simulink model "Mdl4ws_TS8"  (Simulink 5.0)
settings: Solver=ode45  SolverMode=SingleTasking  StartTime=0  StopTime=15  FixedStep=0.002  RelTol=1e-3  AbsTol=1e-6
libraries: Solver_SF x1
settings Model: LastModifiedBy=ywata  ExtModeTrigMode=oneshot  ExtModeArmWhenConnect=off  LimitDataPoints=off  SignalLoggingName=logsout  BlockReductionOpt=off  BooleanDataType=off  RTWTemplateMakefile=grt_vc.tmf  RTWOptions="-aEnforceIntegerDowncast=1 -aFoldNonRolledExpr=1 -aInlineInvariantSignals=0 -aInlineParameters=0 -aLocalBlockOutputs=1 -aRollThreshold=5 -aGenerateReport=0 -aGenCodeOnly=0 -aRTWVerbose=1 -aIncludeHyperlinkInReport=0 -aLaunchReport=0 -aForceParamTrailComments=0 -aGenerateComments=1 -aIgnoreCustomStorageClasses=1 -aIncHierarchyInIds=0 -aMaxRTWIdLen=31 -aShowEliminatedStatements=0 -aPrefixModelToSubsysFcnNames=1 -aIncDataTypeInIds=0 -aInsertBlockDesc=0 -aSimulinkBlockComments=1 -aInlinedPrmAccess=\"Literals\"  -aSuppressErrorStatus=0 -aModelReferenceCompliant=1 -aSupportNonInlinedSFcns=1 -aSupportContinuousTime=1 -aSupportComplex=1 -aSupportNonFinite=1 -aSupportAbsoluteTime=1 -aTargetPreCompLibLocation=\"\" -aTargetLibSuffix=\"\" -aTargetFcnLib=\"ansi_tfl_tmw.mat\" -aMultiInstanceERTCode=0 -aLogVarNameModifier=\"rt_\" -aIsPILTarget=0 -aCombineOutputUpdateFcns=0 -aGenerateASAP2=0 -aGenerateSampleERTMain=0 -aGenerateFullHeader=1 -aUtilityFuncGeneration=\"Auto\" -aIncludeFileDelimiter=\"Auto\" -aIncludeMdlTerminateFcn=1 -aPurelyIntegerCode=0 -aERTCustomFileBanners=0 -aRTWCAPIStates=0 -aRTWCAPIParams=0 -aRTWCAPISignals=0 -aMatFileLogging=1 -aGenFloatMathFcnCalls=\"ANSI_C\" -aExtModeMexFile=\"ext_comm\" -aExtModeTransport=0 -aExtModeStaticAllocSize=1000000 -aExtModeTesting=0 -aExtModeStaticAlloc=0 -aExtMode=0"

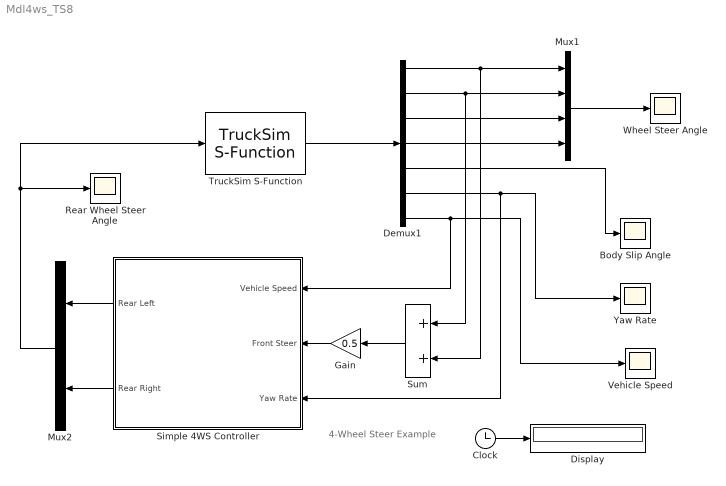
== system Mdl4ws_TS8 ==
  note: 4-Wheel Steer Example
  Body Slip Angle : Scope
      settings: TickLabels=on  YMin=-1  YMax=1.5  DataFormat=Array  Decimation=10
  Clock : Clock
      settings: Decimation=10
  Demux1 : Demux  Outputs=[1 1 1 1 1 1 1]
  Display : Display
      settings: Format=bank  Decimation=100
  Gain : Gain  Orientation=left  Gain=0.5  SaturateOnIntegerOverflow=on
  Mux1 : Mux
  Mux2 : Mux  Orientation=left  Inputs=2
  Rear Wheel Steer Angle : Scope
      settings: TickLabels=on  YMin=-2  YMax=2  DataFormat=Array  Decimation=10
  Simple 4WS Controller : Subsystem  Orientation=left  mask{m=7960, lf=3.102, lr=1.388, Cf=162521, Cr=139081}
      mask prompts: m "body mass (kg)"; lf "length f-G (m)"; lr "length r-G (m)"; Cf "conering power f  (N/rad)"; Cr "conering power r  (N/rad)"
  Sum : Sum  Orientation=left  SaturateOnIntegerOverflow=on  InputSameDT=on
  TruckSim S-Function : Solver_SF/TruckSim S-Function  Priority=1  AncestorBlock=Solver_SF/CarSim S-Function  VehicleCode=???
      settings: AttributesFormatString=Vehicle Code: %<VehicleCode>
  Vehicle Speed : Scope
      settings: TickLabels=on  TimeRange=12  YMin=99.5  YMax=100.5  DataFormat=Array  Decimation=10
  Wheel Steer Angle : Scope
      settings: TickLabels=on  DataFormat=Array  Decimation=10
  Yaw Rate : Scope
      settings: TickLabels=on  YMin=-10  YMax=10  DataFormat=Array  Decimation=10
  wires:
  Sum/1 -> Gain/1
  Gain/1 -> Simple 4WS Controller/2(Front Steer)
  Mux1/1 -> Wheel Steer Angle/1
  Demux1/1 -> Sum/2, Mux1/1
  Demux1/2 -> Sum/1, Mux1/2
  Demux1/3 -> Mux1/3
  Demux1/4 -> Mux1/4
  Demux1/5 -> Body Slip Angle/1
  Demux1/6 -> Simple 4WS Controller/3(Yaw Rate), Yaw Rate/1
  Demux1/7 -> Simple 4WS Controller/1(Vehicle Speed), Vehicle Speed/1
  TruckSim S-Function/1 -> Demux1/1
  Simple 4WS Controller/1(Rear Left) -> Mux2/1
  Simple 4WS Controller/2(Rear Right) -> Mux2/2
  Clock/1 -> Display/1
  Mux2/1 -> Rear Wheel Steer Angle/1, TruckSim S-Function/1

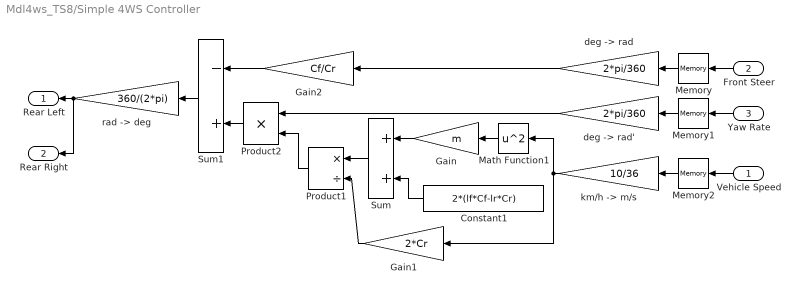
== system Mdl4ws_TS8/Simple 4WS Controller ==
  Vehicle Speed : Inport  Orientation=left
  Front Steer : Inport  Orientation=left  Port=2
  Yaw Rate : Inport  Orientation=left  Port=3
  Constant1 : Constant  Orientation=left  Value=2*(lf*Cf-lr*Cr)
  Gain : Gain  Orientation=left  Gain=m  SaturateOnIntegerOverflow=on
  Gain1 : Gain  Orientation=left  Gain=2*Cr  SaturateOnIntegerOverflow=on
  Gain2 : Gain  Orientation=left  Gain=Cf/Cr  SaturateOnIntegerOverflow=on
  Math Function1 : Math  Orientation=left  Operator=square
  Memory : Memory  Orientation=left
  Memory1 : Memory  Orientation=left
  Memory2 : Memory  Orientation=left  X0=80
  Product1 : Product  Orientation=left  Inputs=*/  RndMeth=Zero  SaturateOnIntegerOverflow=on  InputSameDT=on
  Product2 : Product  Orientation=left  RndMeth=Zero  SaturateOnIntegerOverflow=on  InputSameDT=on
  Sum : Sum  Orientation=left  SaturateOnIntegerOverflow=on  InputSameDT=on
  Sum1 : Sum  Orientation=left  Inputs=-+  SaturateOnIntegerOverflow=on  InputSameDT=on
  "deg -> rad" : Gain  Orientation=left  Gain=2*pi/360  SaturateOnIntegerOverflow=on
  "deg -> rad'" : Gain  Orientation=left  Gain=2*pi/360  SaturateOnIntegerOverflow=on
  "km/h -> m/s" : Gain  Orientation=left  Gain=10/36  SaturateOnIntegerOverflow=on
  "rad -> deg" : Gain  Orientation=left  Gain=360/(2*pi)  SaturateOnIntegerOverflow=on
  Rear Left : Outport  Orientation=left  InitialOutput=0
  Rear Right : Outport  Orientation=left  Port=2  InitialOutput=0
  wires:
  Product1/1 -> Product2/2
  Product2/1 -> Sum1/2
  Gain1/1 -> Product1/2
  Constant1/1 -> Sum/2
  Math Function1/1 -> Gain/1
  Gain/1 -> Sum/1
  Sum/1 -> Product1/1
  Gain2/1 -> Sum1/1
  "km/h -> m/s"/1 -> Math Function1/1, Gain1/1
  "deg -> rad'"/1 -> Product2/1
  "deg -> rad"/1 -> Gain2/1
  Sum1/1 -> "rad -> deg"/1
  Front Steer/1 -> Memory/1
  Memory/1 -> "deg -> rad"/1
  Yaw Rate/1 -> Memory1/1
  Memory1/1 -> "deg -> rad'"/1
  Vehicle Speed/1 -> Memory2/1
  Memory2/1 -> "km/h -> m/s"/1
  "rad -> deg"/1 -> Rear Left/1, Rear Right/1
